simulink model "SMC_seg_tray_atenuacion_chattering_V2"  (R2026b)
settings: Solver=ode4  StopTime=20  FixedStep=0.0001
settings Model: Creator=nestorhernandezcastellanos  LastModifiedBy=nestorhernandezcastellanos

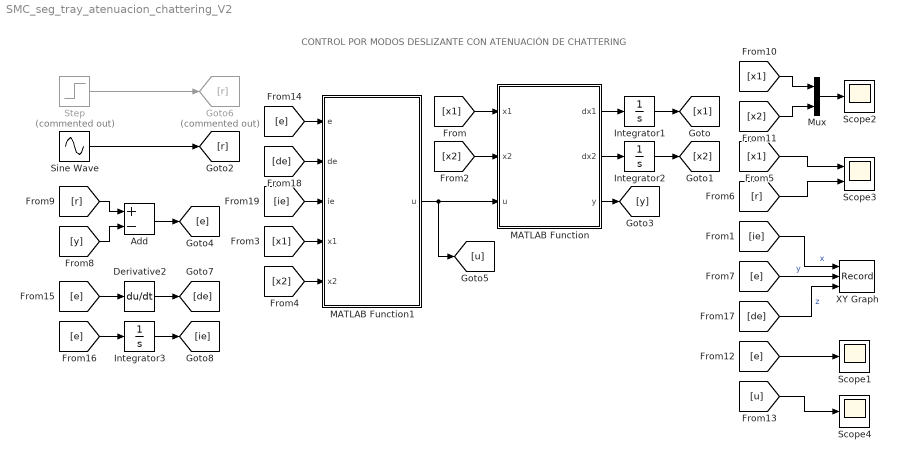
== system SMC_seg_tray_atenuacion_chattering_V2 ==
  note: CONTROL POR MODOS DESLIZANTE CON ATENUACIÓN DE CHATTERING
  Add : Sum  Inputs=+-
  Derivative2 : Derivative
  Goto6 : Goto  Commented=on  GotoTag=r
  Integrator1 : Integrator  InitialCondition=1
  Integrator2 : Integrator  InitialCondition=-2
  Integrator3 : Integrator
  MATLAB Function : MATLAB Function  TreatAsAtomicUnit=on
  MATLAB Function1 : MATLAB Function  TreatAsAtomicUnit=on
  Mux : Mux  Inputs=2
  Scope1 : Scope
      settings: ActiveDisplayYMinimum=-1.1345018827917306  ActiveDisplayYMaximum=0.21051694512557476
  Scope2 : Scope
      settings: ActiveDisplayYMinimum=-2.3780113002128531  ActiveDisplayYMaximum=1.4021017019156774  DataLoggingVariableName=ScopeData2
  Scope3 : Scope  NumInputPorts=2
      settings: ActiveDisplayYMinimum=-1.2500450787630573  ActiveDisplayYMaximum=1.2500253036424773  DataLoggingVariableName=ScopeData3
  Scope4 : Scope
      settings: ActiveDisplayYMinimum=-26.249333606618752  ActiveDisplayYMaximum=26.244002459568783
  Sine Wave : Sin  SampleTime=0
  Step : Step  Commented=on  Time=10  SampleTime=0
  XY Graph : Record  NumPorts=3.0  FileSettingsInternal="{\"entries\":[{\"content\":{\"excelSettings\":{\"content\":{},\"type\":\"Streamout.ExcelSettings\"},\"parquetSettings\":{\"content\":{},\"type\":\"Streamout.ParquetSettings\"}},\"type\":\"Streamout.FileSettingStorage\",\"uuid\":\"\"}],\"packageUris\":[\"http:\\/\\/schema.mathworks.com\\/mf0\\/streamout_blocks\\/R2020a\"],\"version\":\"1.0\"}"  FrameSettings=[0, 0, 0]  Layout=[1 1]  SignalsInternal="{\"entries\":[{\"content\":{\"signals\":[{\"content\":{\"blockPath\":[],\"dimensions\":[1],\"domain\":\"\",\"lineColor\":\"#a2142f\",\"plots\":[ 1 ],\"port\":1,\"sid\":[\"\"],\"signalID\":1,\"signalName\":\"x\"},\"type\":\"RecordBlkView.Signal\",\"uuid\":\"\"},{\"content\":{\"blockPath\":[],\"dimensions\":[1],\"domain\":\"\",\"lineColor\":\"#139fff\",\"plots\":[ 1 ],\"port\":2,\"sid\":[\"\"],\"signalID\":2,\"signalName\":\"y\"},\"type\":\"RecordBlkView.Signal\",\"uuid\":\"\"},{\"content\":{\"blockPath\":[],\"dimensions\":[1],\"domain\":\"\",\"lineColor\":\"#ff6929\",\"lineWidth\":2,\"port\":3,\"sid\":[\"\"],\"signalID\":3,\"signalName\":\"z\"},\"type\":\"RecordBlkView.Signal\",\"uuid\":\"\"}]},\"type\":\"RecordBlkView.InputSignals\",\"uuid\":\"\"}],\"packageUris\":[\"http:\\/\\/schema.mathworks.com\\/mf0\\/streamout_blocks\\/R2020a\"],\"version\":\"1.0\"}"  VisualizationBindings="{\"xyplotplugin\":{\"info\":[{\"series\":[{\"bindingParametersList\":[{\"parameter\":\"X-Axis\",\"signalID\":1,\"signalName\":\"x\"},{\"parameter\":\"Y-Axis\",\"signalID\":2,\"signalName\":\"y\"}],\"seriesID\":0}],\"subplotID\":1}]}}"  CompatibilityTag=XY
  wires:
  MATLAB Function1/1(u) -> [u], MATLAB Function/3(u)
  MATLAB Function/2(dx2) -> Integrator2/1
  MATLAB Function/1(dx1) -> Integrator1/1
  Mux/1 -> Scope2/1
  Sine Wave/1 -> [r]
  [de] -> MATLAB Function1/2(de)
  [x1] -> MATLAB Function/1(x1)
  [ie] -> XY Graph/1  "x"
  [x2] -> MATLAB Function/2(x2)
  [x1] -> MATLAB Function1/4(x1)
  [x2] -> MATLAB Function1/5(x2)
  [x1] -> Scope3/1
  [r] -> Scope3/2
  [e] -> XY Graph/2  "y"
  Integrator2/1 -> [x2]
  Integrator1/1 -> [x1]
  MATLAB Function/3(y) -> [y]
  [y] -> Add/2
  [r] -> Add/1
  [x2] -> Mux/2
  [x1] -> Mux/1
  [e] -> Scope1/1
  [u] -> Scope4/1
  Add/1 -> [e]
  [e] -> MATLAB Function1/1(e)
  Step/1 -> Goto6/1
  [ie] -> MATLAB Function1/3(ie)
  [de] -> XY Graph/3  "z"
  [e] -> Derivative2/1
  [e] -> Integrator3/1
  Integrator3/1 -> [ie]
  Derivative2/1 -> [de]

== matlab function SMC_seg_tray_atenuacion_chattering_V2/MATLAB Function1 ==
  data: e input; de input; ie input; x1 input; x2 input; u output
function u = controlador(e, de, ie, x1, x2)

% Ganancia K>1
K = 3;

% Valor arbitrario positivo
m1 = 2;
m2 = 2.2;
L = 0.8; % Amplitud máxima de mi sistema

Veq = L + m1*abs(x2)+m2*abs(e);
sigma = de + m1*e + m2*ie;
u = K*Veq*sign(sigma);

== matlab function SMC_seg_tray_atenuacion_chattering_V2/MATLAB Function ==
  data: x1 input; x2 input; dx1 output; u input; dx2 output; y output
function [dx1, dx2, y] = planta(x1, x2, u)

dx1 = x2;
dx2 = sin(x1+x2) + cos(x1*x2) + u;

y = x1;
